simulink model "FEAD_BeltDrive"  (R2026a)
settings: Solver=ode23t  StopTime=30  MaxStep=0.01  RelTol=1e-4  AbsTol=1e-6
libraries: fl_lib x42, nesl_utility x28, simulink x1
settings Model: Creator=RICARDO  LastModifiedBy=RICARDO

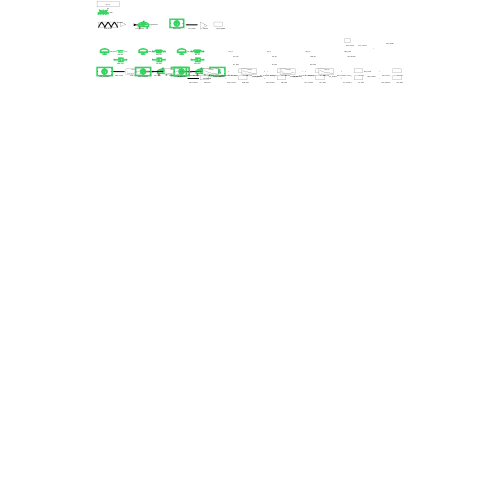
[thumbnail: Simulink's stored preview of the top-level diagram]
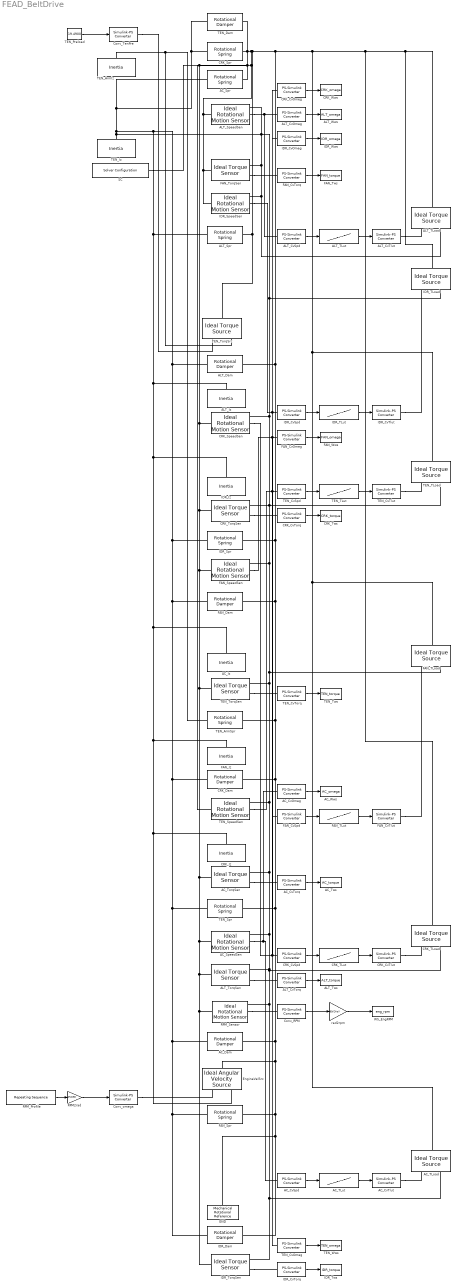
== system FEAD_BeltDrive ==
  AC_CvOmeg : nesl_utility/PS-Simulink Converter  PhysicalDomain=network_engine_domain  SubClassName=ps_output  LeftPortType=input  RightPortType=output  PseudoPeriodic=off  Frequencies=[]  VectorFormat=inherit  Unit=inherit  AffineConversion=off
  AC_CvSpd : nesl_utility/PS-Simulink Converter  PhysicalDomain=network_engine_domain  SubClassName=ps_output  LeftPortType=input  RightPortType=output  PseudoPeriodic=off  Frequencies=[]  VectorFormat=inherit  Unit=inherit  AffineConversion=off
  AC_CvTlut : nesl_utility/Simulink-PS Converter  PhysicalDomain=network_engine_domain  SubClassName=ps_input  LeftPortType=input  RightPortType=output  PseudoPeriodic=off  Frequencies=[]  NoiseDistribution=none  NoiseParameters=[]  Unit=1  AffineConversion=off  FilteringAndDerivatives=provide  SimscapeFilterOrder=1  InputFilterTimeConstant=0.001  UdotUserProvided=0
  AC_CvTorq : nesl_utility/PS-Simulink Converter  PhysicalDomain=network_engine_domain  SubClassName=ps_output  LeftPortType=input  RightPortType=output  PseudoPeriodic=off  Frequencies=[]  VectorFormat=inherit  Unit=inherit  AffineConversion=off
  AC_Dam : fl_lib/Mechanical/Rotational Elements/Rotational Damper  D=22.0300 N*m*s/rad  w_specify=off  w_priority=None  w=0 rad/s  w_nominal_specify=off  w_nominal_value=1  w_nominal_unit=rad/s  t_specify=off  t_priority=None  t=0 N*m  t_nominal_specify=off  t_nominal_value=1  t_nominal_unit=N*m
  AC_Iz : fl_lib/Mechanical/Rotational Elements/Inertia  inertia=0.005516 kg*m^2  num_ports=foundation.enum.numPorts2.one  w_specify=off  w_priority=High  w=0 rad/s  w_nominal_specify=off  w_nominal_value=1  w_nominal_unit=rad/s  t_specify=off  t_priority=None  t=0 N*m  t_nominal_specify=off  t_nominal_value=1  t_nominal_unit=N*m
  AC_SpeedSen : fl_lib/Mechanical/Mechanical Sensors/Ideal Rotational Motion Sensor  reference=foundation.enum.MeasurementReference.difference  acceleration_port=false  velocity_port=true  position_port=true  wrap_angle=false  offset=0 rad
  AC_Spr : fl_lib/Mechanical/Rotational Elements/Rotational Spring  spr_rate=4405.99 N*m/rad  w_specify=off  w_priority=None  w=0 rad/s  w_nominal_specify=off  w_nominal_value=1  w_nominal_unit=rad/s  t_specify=off  t_priority=None  t=0 N*m  t_nominal_specify=off  t_nominal_value=1  t_nominal_unit=N*m  phi_specify=off  phi_priority=High  phi=0 rad  phi_nominal_specify=off  phi_nominal_value=1  phi_nominal_unit=rad
  AC_TLoad : fl_lib/Mechanical/Mechanical Sources/Ideal Torque Source
  AC_TLut : Lookup_n-D  NumberOfTableDimensions=1  BreakpointsForDimension1=[52.3599 83.7758 104.72 125.664 146.608 167.552 188.496 209.44]  Table=[19.0986 15.8757 16.5203 16.7113 16.5066 16.7113 17.4009 17.3797]  ExtrapMethod=Clip  InternalRulePriority=Speed  RndMeth=Simplest
  AC_TorqSen : fl_lib/Mechanical/Mechanical Sensors/Ideal Torque Sensor
  AC_Tws : ToWorkspace  VariableName=AC_torque  SampleTime=-1
  AC_Wws : ToWorkspace  VariableName=AC_omega  SampleTime=-1
  ALT_CvOmeg : nesl_utility/PS-Simulink Converter  PhysicalDomain=network_engine_domain  SubClassName=ps_output  LeftPortType=input  RightPortType=output  PseudoPeriodic=off  Frequencies=[]  VectorFormat=inherit  Unit=inherit  AffineConversion=off
  ALT_CvSpd : nesl_utility/PS-Simulink Converter  PhysicalDomain=network_engine_domain  SubClassName=ps_output  LeftPortType=input  RightPortType=output  PseudoPeriodic=off  Frequencies=[]  VectorFormat=inherit  Unit=inherit  AffineConversion=off
  ALT_CvTlut : nesl_utility/Simulink-PS Converter  PhysicalDomain=network_engine_domain  SubClassName=ps_input  LeftPortType=input  RightPortType=output  PseudoPeriodic=off  Frequencies=[]  NoiseDistribution=none  NoiseParameters=[]  Unit=1  AffineConversion=off  FilteringAndDerivatives=provide  SimscapeFilterOrder=1  InputFilterTimeConstant=0.001  UdotUserProvided=0
  ALT_CvTorq : nesl_utility/PS-Simulink Converter  PhysicalDomain=network_engine_domain  SubClassName=ps_output  LeftPortType=input  RightPortType=output  PseudoPeriodic=off  Frequencies=[]  VectorFormat=inherit  Unit=inherit  AffineConversion=off
  ALT_Dam : fl_lib/Mechanical/Rotational Elements/Rotational Damper  D=4.4114 N*m*s/rad  w_specify=off  w_priority=None  w=0 rad/s  w_nominal_specify=off  w_nominal_value=1  w_nominal_unit=rad/s  t_specify=off  t_priority=None  t=0 N*m  t_nominal_specify=off  t_nominal_value=1  t_nominal_unit=N*m
  ALT_Iz : fl_lib/Mechanical/Rotational Elements/Inertia  inertia=0.000543 kg*m^2  num_ports=foundation.enum.numPorts2.one  w_specify=off  w_priority=High  w=0 rad/s  w_nominal_specify=off  w_nominal_value=1  w_nominal_unit=rad/s  t_specify=off  t_priority=None  t=0 N*m  t_nominal_specify=off  t_nominal_value=1  t_nominal_unit=N*m
  ALT_SpeedSen : fl_lib/Mechanical/Mechanical Sensors/Ideal Rotational Motion Sensor  reference=foundation.enum.MeasurementReference.difference  acceleration_port=false  velocity_port=true  position_port=true  wrap_angle=false  offset=0 rad
  ALT_Spr : fl_lib/Mechanical/Rotational Elements/Rotational Spring  spr_rate=882.29 N*m/rad  w_specify=off  w_priority=None  w=0 rad/s  w_nominal_specify=off  w_nominal_value=1  w_nominal_unit=rad/s  t_specify=off  t_priority=None  t=0 N*m  t_nominal_specify=off  t_nominal_value=1  t_nominal_unit=N*m  phi_specify=off  phi_priority=High  phi=0 rad  phi_nominal_specify=off  phi_nominal_value=1  phi_nominal_unit=rad
  ALT_TLoad : fl_lib/Mechanical/Mechanical Sources/Ideal Torque Source
  ALT_TLut : Lookup_n-D  NumberOfTableDimensions=1  BreakpointsForDimension1=[52.3599 83.7758 104.72 125.664 146.608 167.552 188.496 209.44]  Table=[30.5577 25.3056 25.4966 24.3507 22.0316 20.2923 18.8333 17.6662]  ExtrapMethod=Clip  InternalRulePriority=Speed  RndMeth=Simplest
  ALT_TorqSen : fl_lib/Mechanical/Mechanical Sensors/Ideal Torque Sensor
  ALT_Tws : ToWorkspace  VariableName=ALT_torque  SampleTime=-1
  ALT_Wws : ToWorkspace  VariableName=ALT_omega  SampleTime=-1
  CRK_CvOmeg : nesl_utility/PS-Simulink Converter  PhysicalDomain=network_engine_domain  SubClassName=ps_output  LeftPortType=input  RightPortType=output  PseudoPeriodic=off  Frequencies=[]  VectorFormat=inherit  Unit=inherit  AffineConversion=off
  CRK_CvSpd : nesl_utility/PS-Simulink Converter  PhysicalDomain=network_engine_domain  SubClassName=ps_output  LeftPortType=input  RightPortType=output  PseudoPeriodic=off  Frequencies=[]  VectorFormat=inherit  Unit=inherit  AffineConversion=off
  CRK_CvTlut : nesl_utility/Simulink-PS Converter  PhysicalDomain=network_engine_domain  SubClassName=ps_input  LeftPortType=input  RightPortType=output  PseudoPeriodic=off  Frequencies=[]  NoiseDistribution=none  NoiseParameters=[]  Unit=1  AffineConversion=off  FilteringAndDerivatives=provide  SimscapeFilterOrder=1  InputFilterTimeConstant=0.001  UdotUserProvided=0
  CRK_CvTorq : nesl_utility/PS-Simulink Converter  PhysicalDomain=network_engine_domain  SubClassName=ps_output  LeftPortType=input  RightPortType=output  PseudoPeriodic=off  Frequencies=[]  VectorFormat=inherit  Unit=inherit  AffineConversion=off
  CRK_Dam : fl_lib/Mechanical/Rotational Elements/Rotational Damper  D=26.6791 N*m*s/rad  w_specify=off  w_priority=None  w=0 rad/s  w_nominal_specify=off  w_nominal_value=1  w_nominal_unit=rad/s  t_specify=off  t_priority=None  t=0 N*m  t_nominal_specify=off  t_nominal_value=1  t_nominal_unit=N*m
  CRK_Iz : fl_lib/Mechanical/Rotational Elements/Inertia  inertia=0.013296 kg*m^2  num_ports=foundation.enum.numPorts2.one  w_specify=off  w_priority=High  w=0 rad/s  w_nominal_specify=off  w_nominal_value=1  w_nominal_unit=rad/s  t_specify=off  t_priority=None  t=0 N*m  t_nominal_specify=off  t_nominal_value=1  t_nominal_unit=N*m
  CRK_SpeedSen : fl_lib/Mechanical/Mechanical Sensors/Ideal Rotational Motion Sensor  reference=foundation.enum.MeasurementReference.difference  acceleration_port=false  velocity_port=true  position_port=true  wrap_angle=false  offset=0 rad
  CRK_Spr : fl_lib/Mechanical/Rotational Elements/Rotational Spring  spr_rate=5335.83 N*m/rad  w_specify=off  w_priority=None  w=0 rad/s  w_nominal_specify=off  w_nominal_value=1  w_nominal_unit=rad/s  t_specify=off  t_priority=None  t=0 N*m  t_nominal_specify=off  t_nominal_value=1  t_nominal_unit=N*m  phi_specify=off  phi_priority=High  phi=0 rad  phi_nominal_specify=off  phi_nominal_value=1  phi_nominal_unit=rad
  CRK_TLoad : fl_lib/Mechanical/Mechanical Sources/Ideal Torque Source
  CRK_TLut : Lookup_n-D  NumberOfTableDimensions=1  BreakpointsForDimension1=[52.3599 83.7758 104.72 125.664 146.608 167.552 188.496 209.44]  Table=[63.0254 54.3116 62.4524 66.5268 72.9157 78.7817 96.3948 106.188]  ExtrapMethod=Clip  InternalRulePriority=Speed  RndMeth=Simplest
  CRK_TorqSen : fl_lib/Mechanical/Mechanical Sensors/Ideal Torque Sensor
  CRK_Tws : ToWorkspace  VariableName=CRK_torque  SampleTime=-1
  CRK_Wws : ToWorkspace  VariableName=CRK_omega  SampleTime=-1
  Conv_RPM : nesl_utility/PS-Simulink Converter  PhysicalDomain=network_engine_domain  SubClassName=ps_output  LeftPortType=input  RightPortType=output  PseudoPeriodic=off  Frequencies=[]  VectorFormat=inherit  Unit=inherit  AffineConversion=off
  Conv_TenPre : nesl_utility/Simulink-PS Converter  PhysicalDomain=network_engine_domain  SubClassName=ps_input  LeftPortType=input  RightPortType=output  PseudoPeriodic=off  Frequencies=[]  NoiseDistribution=none  NoiseParameters=[]  Unit=1  AffineConversion=off  FilteringAndDerivatives=provide  SimscapeFilterOrder=1  InputFilterTimeConstant=0.001  UdotUserProvided=0
  Conv_omega : nesl_utility/Simulink-PS Converter  PhysicalDomain=network_engine_domain  SubClassName=ps_input  LeftPortType=input  RightPortType=output  PseudoPeriodic=off  Frequencies=[]  NoiseDistribution=none  NoiseParameters=[]  Unit=1  AffineConversion=off  FilteringAndDerivatives=provide  SimscapeFilterOrder=1  InputFilterTimeConstant=0.001  UdotUserProvided=0
  EngineVelSrc : fl_lib/Mechanical/Mechanical Sources/Ideal Angular Velocity Source
  FAN_CvOmeg : nesl_utility/PS-Simulink Converter  PhysicalDomain=network_engine_domain  SubClassName=ps_output  LeftPortType=input  RightPortType=output  PseudoPeriodic=off  Frequencies=[]  VectorFormat=inherit  Unit=inherit  AffineConversion=off
  FAN_CvSpd : nesl_utility/PS-Simulink Converter  PhysicalDomain=network_engine_domain  SubClassName=ps_output  LeftPortType=input  RightPortType=output  PseudoPeriodic=off  Frequencies=[]  VectorFormat=inherit  Unit=inherit  AffineConversion=off
  FAN_CvTlut : nesl_utility/Simulink-PS Converter  PhysicalDomain=network_engine_domain  SubClassName=ps_input  LeftPortType=input  RightPortType=output  PseudoPeriodic=off  Frequencies=[]  NoiseDistribution=none  NoiseParameters=[]  Unit=1  AffineConversion=off  FilteringAndDerivatives=provide  SimscapeFilterOrder=1  InputFilterTimeConstant=0.001  UdotUserProvided=0
  FAN_CvTorq : nesl_utility/PS-Simulink Converter  PhysicalDomain=network_engine_domain  SubClassName=ps_output  LeftPortType=input  RightPortType=output  PseudoPeriodic=off  Frequencies=[]  VectorFormat=inherit  Unit=inherit  AffineConversion=off
  FAN_Dam : fl_lib/Mechanical/Rotational Elements/Rotational Damper  D=25.3764 N*m*s/rad  w_specify=off  w_priority=None  w=0 rad/s  w_nominal_specify=off  w_nominal_value=1  w_nominal_unit=rad/s  t_specify=off  t_priority=None  t=0 N*m  t_nominal_specify=off  t_nominal_value=1  t_nominal_unit=N*m
  FAN_Iz : fl_lib/Mechanical/Rotational Elements/Inertia  inertia=0.015553 kg*m^2  num_ports=foundation.enum.numPorts2.one  w_specify=off  w_priority=High  w=0 rad/s  w_nominal_specify=off  w_nominal_value=1  w_nominal_unit=rad/s  t_specify=off  t_priority=None  t=0 N*m  t_nominal_specify=off  t_nominal_value=1  t_nominal_unit=N*m
  FAN_SpeedSen : fl_lib/Mechanical/Mechanical Sensors/Ideal Rotational Motion Sensor  reference=foundation.enum.MeasurementReference.difference  acceleration_port=false  velocity_port=true  position_port=true  wrap_angle=false  offset=0 rad
  FAN_Spr : fl_lib/Mechanical/Rotational Elements/Rotational Spring  spr_rate=5075.28 N*m/rad  w_specify=off  w_priority=None  w=0 rad/s  w_nominal_specify=off  w_nominal_value=1  w_nominal_unit=rad/s  t_specify=off  t_priority=None  t=0 N*m  t_nominal_specify=off  t_nominal_value=1  t_nominal_unit=N*m  phi_specify=off  phi_priority=High  phi=0 rad  phi_nominal_specify=off  phi_nominal_value=1  phi_nominal_unit=rad
  FAN_TLoad : fl_lib/Mechanical/Mechanical Sources/Ideal Torque Source
  FAN_TLut : Lookup_n-D  NumberOfTableDimensions=1  BreakpointsForDimension1=[52.3599 83.7758 104.72 125.664 146.608 167.552 188.496 209.44]  Table=[9.5493 9.5493 17.1887 22.2817 31.3763 38.794 57.2958 68.2775]  ExtrapMethod=Clip  InternalRulePriority=Speed  RndMeth=Simplest
  FAN_TorqSen : fl_lib/Mechanical/Mechanical Sensors/Ideal Torque Sensor
  FAN_Tws : ToWorkspace  VariableName=FAN_torque  SampleTime=-1
  FAN_Wws : ToWorkspace  VariableName=FAN_omega  SampleTime=-1
  GND : fl_lib/Mechanical/Rotational Elements/Mechanical Rotational Reference
  IDR_CvOmeg : nesl_utility/PS-Simulink Converter  PhysicalDomain=network_engine_domain  SubClassName=ps_output  LeftPortType=input  RightPortType=output  PseudoPeriodic=off  Frequencies=[]  VectorFormat=inherit  Unit=inherit  AffineConversion=off
  IDR_CvSpd : nesl_utility/PS-Simulink Converter  PhysicalDomain=network_engine_domain  SubClassName=ps_output  LeftPortType=input  RightPortType=output  PseudoPeriodic=off  Frequencies=[]  VectorFormat=inherit  Unit=inherit  AffineConversion=off
  IDR_CvTlut : nesl_utility/Simulink-PS Converter  PhysicalDomain=network_engine_domain  SubClassName=ps_input  LeftPortType=input  RightPortType=output  PseudoPeriodic=off  Frequencies=[]  NoiseDistribution=none  NoiseParameters=[]  Unit=1  AffineConversion=off  FilteringAndDerivatives=provide  SimscapeFilterOrder=1  InputFilterTimeConstant=0.001  UdotUserProvided=0
  IDR_CvTorq : nesl_utility/PS-Simulink Converter  PhysicalDomain=network_engine_domain  SubClassName=ps_output  LeftPortType=input  RightPortType=output  PseudoPeriodic=off  Frequencies=[]  VectorFormat=inherit  Unit=inherit  AffineConversion=off
  IDR_Dam : fl_lib/Mechanical/Rotational Elements/Rotational Damper  D=7.0276 N*m*s/rad  w_specify=off  w_priority=None  w=0 rad/s  w_nominal_specify=off  w_nominal_value=1  w_nominal_unit=rad/s  t_specify=off  t_priority=None  t=0 N*m  t_nominal_specify=off  t_nominal_value=1  t_nominal_unit=N*m
  IDR_Iz : fl_lib/Mechanical/Rotational Elements/Inertia  inertia=0.000599 kg*m^2  num_ports=foundation.enum.numPorts2.one  w_specify=off  w_priority=High  w=0 rad/s  w_nominal_specify=off  w_nominal_value=1  w_nominal_unit=rad/s  t_specify=off  t_priority=None  t=0 N*m  t_nominal_specify=off  t_nominal_value=1  t_nominal_unit=N*m
  IDR_SpeedSen : fl_lib/Mechanical/Mechanical Sensors/Ideal Rotational Motion Sensor  reference=foundation.enum.MeasurementReference.difference  acceleration_port=false  velocity_port=true  position_port=true  wrap_angle=false  offset=0 rad
  IDR_Spr : fl_lib/Mechanical/Rotational Elements/Rotational Spring  spr_rate=1405.53 N*m/rad  w_specify=off  w_priority=None  w=0 rad/s  w_nominal_specify=off  w_nominal_value=1  w_nominal_unit=rad/s  t_specify=off  t_priority=None  t=0 N*m  t_nominal_specify=off  t_nominal_value=1  t_nominal_unit=N*m  phi_specify=off  phi_priority=High  phi=0 rad  phi_nominal_specify=off  phi_nominal_value=1  phi_nominal_unit=rad
  IDR_TLoad : fl_lib/Mechanical/Mechanical Sources/Ideal Torque Source
  IDR_TLut : Lookup_n-D  NumberOfTableDimensions=1  BreakpointsForDimension1=[52.3599 83.7758 104.72 125.664 146.608 167.552 188.496 209.44]  Table=[1.90986 1.79049 1.62338 1.59155 1.5006 1.49208 1.43239 1.43239]  ExtrapMethod=Clip  InternalRulePriority=Speed  RndMeth=Simplest
  IDR_TorqSen : fl_lib/Mechanical/Mechanical Sensors/Ideal Torque Sensor
  IDR_Tws : ToWorkspace  VariableName=IDR_torque  SampleTime=-1
  IDR_Wws : ToWorkspace  VariableName=IDR_omega  SampleTime=-1
  RPM2rad : Gain  Gain=2*pi/60
  RPM_Profile : simulink/Sources/Repeating Sequence  rep_seq_t="[0  5   15   25   30]"  rep_seq_y=[600 1200 2000 1200 600]
  RPM_Sensor : fl_lib/Mechanical/Mechanical Sensors/Ideal Rotational Motion Sensor  reference=foundation.enum.MeasurementReference.difference  acceleration_port=false  velocity_port=true  position_port=true  wrap_angle=false  offset=0 rad
  SC : nesl_utility/Solver Configuration  PhysicalDomain=network_engine_domain  SubClassName=solver  LeftPortType=input  RightPortType=generic  Tones=[]  Harmonics=[]  SimulateNoise=off  Profile=off  UseLocalSampling=off  EnableSwitchedLinearOptims=on  FrequencyDomain=off  UseCCode=off  RelTol=0.001  AbsTol=0.001  MinStep=1e-09  ToWorkspace=off  RevertToSquareIcSolve=off  NumHomotopyIterations=100  PhasorMode=off  PhasorModeNumHarmonics=1  ConsistencySolver=NEWTON_XTOL_AFTER_FTOL  CanonicalOrdering=CANONICAL  OptimizeIntermediates=OPTIMIZED  IndexReductionMethod=DerivativeReplacement  DoDC=off  ResidualTolerance=1e-09  ConsistencyTolSource=GLOBAL  ConsistencyAbsTol=0.001  ConsistencyRelTol=0.001  ConsistencyTolFactor=0.001  UseLocalSolver=off  LocalSolverChoice=NE_BACKWARD_EULER_ADVANCER  ResolveIndetEquations=on  FunctionEvalNumThread=1  LocalSolverSampleTime=0.001  DoFixedCost=off  MaxNonlinIter=3  MaxModeIter=2  ComputeImpulses=off  ImpulseIterations=2  LinearAlgebra=auto  LinearAlgebraNumThread=0  EquationFormulation=NE_TIME_EF  DelaysMemoryBudget=1024  AutomaticFiltering=on  FilteringTimeConstant=0.001  PartitionStorageMethod=AS_NEEDED  PartitionMemoryBudget=1024  PartitionMethod=ROBUST  MultibodyUseLocalSolver=off  MultibodyLocalSolverChoice=ODE1  MultibodyLocalSolverSampleTime=0.001
  TEN_ArmIz : fl_lib/Mechanical/Rotational Elements/Inertia  inertia=0.00500 kg*m^2  num_ports=foundation.enum.numPorts2.one  w_specify=off  w_priority=High  w=0 rad/s  w_nominal_specify=off  w_nominal_value=1  w_nominal_unit=rad/s  t_specify=off  t_priority=None  t=0 N*m  t_nominal_specify=off  t_nominal_value=1  t_nominal_unit=N*m
  TEN_ArmSpr : fl_lib/Mechanical/Rotational Elements/Rotational Spring  spr_rate=0.8830 N*m/rad  w_specify=off  w_priority=None  w=0 rad/s  w_nominal_specify=off  w_nominal_value=1  w_nominal_unit=rad/s  t_specify=off  t_priority=None  t=0 N*m  t_nominal_specify=off  t_nominal_value=1  t_nominal_unit=N*m  phi_specify=off  phi_priority=High  phi=0 rad  phi_nominal_specify=off  phi_nominal_value=1  phi_nominal_unit=rad
  TEN_CvOmeg : nesl_utility/PS-Simulink Converter  PhysicalDomain=network_engine_domain  SubClassName=ps_output  LeftPortType=input  RightPortType=output  PseudoPeriodic=off  Frequencies=[]  VectorFormat=inherit  Unit=inherit  AffineConversion=off
  TEN_CvSpd : nesl_utility/PS-Simulink Converter  PhysicalDomain=network_engine_domain  SubClassName=ps_output  LeftPortType=input  RightPortType=output  PseudoPeriodic=off  Frequencies=[]  VectorFormat=inherit  Unit=inherit  AffineConversion=off
  TEN_CvTlut : nesl_utility/Simulink-PS Converter  PhysicalDomain=network_engine_domain  SubClassName=ps_input  LeftPortType=input  RightPortType=output  PseudoPeriodic=off  Frequencies=[]  NoiseDistribution=none  NoiseParameters=[]  Unit=1  AffineConversion=off  FilteringAndDerivatives=provide  SimscapeFilterOrder=1  InputFilterTimeConstant=0.001  UdotUserProvided=0
  TEN_CvTorq : nesl_utility/PS-Simulink Converter  PhysicalDomain=network_engine_domain  SubClassName=ps_output  LeftPortType=input  RightPortType=output  PseudoPeriodic=off  Frequencies=[]  VectorFormat=inherit  Unit=inherit  AffineConversion=off
  TEN_Dam : fl_lib/Mechanical/Rotational Elements/Rotational Damper  D=7.4538 N*m*s/rad  w_specify=off  w_priority=None  w=0 rad/s  w_nominal_specify=off  w_nominal_value=1  w_nominal_unit=rad/s  t_specify=off  t_priority=None  t=0 N*m  t_nominal_specify=off  t_nominal_value=1  t_nominal_unit=N*m
  TEN_Iz : fl_lib/Mechanical/Rotational Elements/Inertia  inertia=0.000674 kg*m^2  num_ports=foundation.enum.numPorts2.one  w_specify=off  w_priority=High  w=0 rad/s  w_nominal_specify=off  w_nominal_value=1  w_nominal_unit=rad/s  t_specify=off  t_priority=None  t=0 N*m  t_nominal_specify=off  t_nominal_value=1  t_nominal_unit=N*m
  TEN_Preload : Constant  Value=19.4900
  TEN_SpeedSen : fl_lib/Mechanical/Mechanical Sensors/Ideal Rotational Motion Sensor  reference=foundation.enum.MeasurementReference.difference  acceleration_port=false  velocity_port=true  position_port=true  wrap_angle=false  offset=0 rad
  TEN_Spr : fl_lib/Mechanical/Rotational Elements/Rotational Spring  spr_rate=1490.77 N*m/rad  w_specify=off  w_priority=None  w=0 rad/s  w_nominal_specify=off  w_nominal_value=1  w_nominal_unit=rad/s  t_specify=off  t_priority=None  t=0 N*m  t_nominal_specify=off  t_nominal_value=1  t_nominal_unit=N*m  phi_specify=off  phi_priority=High  phi=0 rad  phi_nominal_specify=off  phi_nominal_value=1  phi_nominal_unit=rad
  TEN_TLoad : fl_lib/Mechanical/Mechanical Sources/Ideal Torque Source
  TEN_TLut : Lookup_n-D  NumberOfTableDimensions=1  BreakpointsForDimension1=[52.3599 83.7758 104.72 125.664 146.608 167.552 188.496 209.44]  Table=[1.90986 1.79049 1.62338 1.59155 1.5006 1.49208 1.43239 1.28916]  ExtrapMethod=Clip  InternalRulePriority=Speed  RndMeth=Simplest
  TEN_TorqSen : fl_lib/Mechanical/Mechanical Sensors/Ideal Torque Sensor
  TEN_TorqSrc : fl_lib/Mechanical/Mechanical Sources/Ideal Torque Source
  TEN_Tws : ToWorkspace  VariableName=TEN_torque  SampleTime=-1
  TEN_Wws : ToWorkspace  VariableName=TEN_omega  SampleTime=-1
  WS_EngRPM : ToWorkspace  VariableName=eng_rpm  SampleTime=-1
  rad2rpm : Gain  Gain=60/(2*pi)
  wires:
  RPM_Profile/1 -> RPM2rad/1
  TEN_Preload/1 -> Conv_TenPre/1
  RPM2rad/1 -> Conv_omega/1
  rad2rpm/1 -> WS_EngRPM/1
  IDR_TLut/1 -> IDR_CvTlut/1
  IDR_CvTorq/1 -> IDR_Tws/1
  ALT_TLut/1 -> ALT_CvTlut/1
  CRK_CvOmeg/1 -> CRK_Wws/1
  ALT_CvOmeg/1 -> ALT_Wws/1
  ALT_CvTorq/1 -> ALT_Tws/1
  IDR_CvOmeg/1 -> IDR_Wws/1
  Conv_RPM/1 -> rad2rpm/1
  FAN_CvTorq/1 -> FAN_Tws/1
  ALT_CvSpd/1 -> ALT_TLut/1
  IDR_CvSpd/1 -> IDR_TLut/1
  FAN_CvOmeg/1 -> FAN_Wws/1
  TEN_CvSpd/1 -> TEN_TLut/1
  CRK_TLut/1 -> CRK_CvTlut/1
  CRK_CvTorq/1 -> CRK_Tws/1
  TEN_CvTorq/1 -> TEN_Tws/1
  AC_CvOmeg/1 -> AC_Wws/1
  FAN_CvSpd/1 -> FAN_TLut/1
  AC_TLut/1 -> AC_CvTlut/1
  AC_CvTorq/1 -> AC_Tws/1
  CRK_CvSpd/1 -> CRK_TLut/1
  AC_CvSpd/1 -> AC_TLut/1
  TEN_CvOmeg/1 -> TEN_Wws/1
  TEN_TLut/1 -> TEN_CvTlut/1
  FAN_TLut/1 -> FAN_CvTlut/1
  connections:
  Conv_omega/RConn1 -- EngineVelSrc/RConn1
  ALT_SpeedSen/RConn2 -- ALT_CvOmeg/LConn1 -- ALT_CvSpd/LConn1
  TEN_ArmIz/LConn1 -- TEN_ArmSpr/LConn1 -- TEN_TorqSrc/RConn2
  AC_SpeedSen/RConn2 -- AC_CvOmeg/LConn1 -- AC_CvSpd/LConn1
  Conv_TenPre/RConn1 -- TEN_TorqSrc/RConn1
  TEN_Iz/LConn1 -- IDR_SpeedSen/RConn1 -- ALT_TLoad/RConn2 -- FAN_TorqSen/RConn1 -- IDR_TorqSen/RConn1 -- AC_TLoad/RConn2 -- RPM_Sensor/RConn1 -- CRK_TLoad/RConn2 -- ALT_TorqSen/RConn1 -- AC_SpeedSen/RConn1 -- AC_TorqSen/RConn1 -- TEN_SpeedSen/RConn1 -- TEN_TorqSen/RConn1 -- FAN_TLoad/RConn2 -- FAN_SpeedSen/RConn1 -- TEN_TLoad/RConn2 -- CRK_TorqSen/RConn1 -- CRK_SpeedSen/RConn1 -- IDR_TLoad/RConn2 -- ALT_SpeedSen/RConn1 -- EngineVelSrc/RConn2 -- CRK_Iz/LConn1 -- FAN_Iz/LConn1 -- AC_Iz/LConn1 -- IDR_Iz/LConn1 -- ALT_Iz/LConn1 -- ALT_Spr/LConn1 -- FAN_Spr/LConn1 -- IDR_Dam/LConn1 -- AC_Dam/LConn1 -- TEN_Spr/LConn1 -- CRK_Dam/LConn1 -- FAN_Dam/LConn1 -- IDR_Spr/LConn1 -- ALT_Dam/LConn1 -- CRK_Spr/LConn1 -- TEN_Dam/LConn1 -- AC_Spr/LConn1
  SC/RConn1 -- IDR_TorqSen/LConn1 -- RPM_Sensor/LConn1 -- ALT_TorqSen/LConn1 -- AC_SpeedSen/LConn1 -- AC_TorqSen/LConn1 -- TEN_TorqSen/LConn1 -- FAN_SpeedSen/LConn1 -- CRK_TorqSen/LConn1 -- CRK_SpeedSen/LConn1 -- FAN_TorqSen/LConn1 -- IDR_SpeedSen/LConn1 -- ALT_SpeedSen/LConn1 -- TEN_TorqSrc/LConn1 -- ALT_Spr/RConn1 -- IDR_Dam/RConn1 -- GND/LConn1 -- FAN_Spr/RConn1 -- EngineVelSrc/LConn1 -- AC_Dam/RConn1 -- TEN_Spr/RConn1 -- CRK_Dam/RConn1 -- TEN_ArmSpr/RConn1 -- FAN_Dam/RConn1 -- IDR_Spr/RConn1 -- ALT_Dam/RConn1 -- FAN_TLoad/LConn1 -- AC_TLoad/LConn1 -- TEN_TLoad/LConn1 -- ALT_TLoad/LConn1 -- IDR_TLoad/LConn1 -- CRK_TLoad/LConn1 -- TEN_SpeedSen/LConn1 -- AC_Spr/RConn1 -- TEN_Dam/RConn1 -- CRK_Spr/RConn1
  FAN_TorqSen/RConn2 -- FAN_CvTorq/LConn1
  IDR_SpeedSen/RConn2 -- IDR_CvSpd/LConn1 -- IDR_CvOmeg/LConn1
  CRK_SpeedSen/RConn2 -- CRK_CvSpd/LConn1 -- CRK_CvOmeg/LConn1
  CRK_TorqSen/RConn2 -- CRK_CvTorq/LConn1
  FAN_SpeedSen/RConn2 -- FAN_CvSpd/LConn1 -- FAN_CvOmeg/LConn1
  TEN_TorqSen/RConn2 -- TEN_CvTorq/LConn1
  TEN_SpeedSen/RConn2 -- TEN_CvSpd/LConn1 -- TEN_CvOmeg/LConn1
  AC_TorqSen/RConn2 -- AC_CvTorq/LConn1
  ALT_TorqSen/RConn2 -- ALT_CvTorq/LConn1
  RPM_Sensor/RConn2 -- Conv_RPM/LConn1
  IDR_TorqSen/RConn2 -- IDR_CvTorq/LConn1
  FAN_CvTlut/RConn1 -- FAN_TLoad/RConn1
  ALT_CvTlut/RConn1 -- ALT_TLoad/RConn1
  IDR_CvTlut/RConn1 -- IDR_TLoad/RConn1
  TEN_CvTlut/RConn1 -- TEN_TLoad/RConn1
  CRK_CvTlut/RConn1 -- CRK_TLoad/RConn1
  AC_CvTlut/RConn1 -- AC_TLoad/RConn1
